simulink model "motor1"  (R2016a)
settings: Solver=ode3  StartTime=0.0  StopTime=1  MaxStep=1e-4  RelTol=1e-3
values from neighbouring files (symbols this model uses):
  D = chromosome(chromosomeProperties.populationNumber+1).gene(3).value    [HW1.m]    (also in motorModel01.m = 0.03; motorModel03.m = 8.42)
  I = chromosome(chromosomeProperties.populationNumber+1).gene(2).value    [HW1.m]    (also in motorModel01.m = 14.2; motorModel03.m = 18638)
  P = chromosome(chromosomeProperties.populationNumber+1).gene(1).value    [HW1.m]    (also in motorModel01.m = 1.35; motorModel03.m = 792.12)
libraries: simulink x1
settings Model: Creator=Minh  LastModifiedBy=Minh
settings DataIOCC: LimitDataPoints=on  SaveFormat=Array
settings DebuggingCC: UnderspecifiedInitializationDetection=Classic  MergeDetectMultiDrivingBlocksExec=none  SolverPrmCheckMsg=warning  StateNameClashWarn=warning
settings HardwareCC: ProdBitPerPointer=32  ProdLargestAtomicFloat=None  ProdIntDivRoundTo=Undefined  ProdEndianess=Unspecified  ProdWordSize=32  ProdHWDeviceType=32-bit Generic
settings ModelReferenceCC: PropagateSignalLabelsOutOfModel=off
settings ConfigComp: CovModelRefEnable=Off
settings ConfigurationSet: Description=SimMechanics 2G

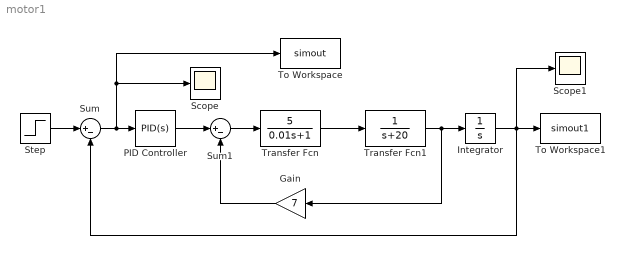
== system motor1 ==
  Gain : Gain  Gain=7
  Integrator : Integrator
  PID Controller : simulink/Continuous/PID Controller  Controller=PID  TimeDomain=Continuous-time  SampleTime=-1  IntegratorMethod=Forward Euler  FilterMethod=Forward Euler  Form=Parallel  UseFilter=on  ControllerParametersSource=internal  P=P  I=I  D=D  N=1000  InitialConditionSource=internal  InitialConditionForIntegrator=0  InitialConditionForFilter=0  ExternalReset=none  LimitOutput=off  UpperSaturationLimit=inf  LowerSaturationLimit=-inf  LinearizeAsGain=on  AntiWindupMode=none  Kb=1  TrackingMode=off  Kt=1  PParamMin=[]  PParamMax=[]  IParamMin=[]  IParamMax=[]  DParamMin=[]  DParamMax=[]  NParamMin=[]  NParamMax=[]  KbParamMin=[]  KbParamMax=[]  KtParamMin=[]  KtParamMax=[]  POutMin=[]  POutMax=[]  IOutMin=[]  IOutMax=[]  DOutMin=[]  DOutMax=[]  NOutMin=[]  NOutMax=[]  KbOutMin=[]  KbOutMax=[]  KtOutMin=[]  KtOutMax=[]  IntegratorOutMin=[]  IntegratorOutMax=[]  FilterOutMin=[]  FilterOutMax=[]  SumOutMin=[]  SumOutMax=[]  SumI1OutMin=[]  SumI1OutMax=[]  SumI2OutMin=[]  SumI2OutMax=[]  SumI3OutMin=[]  SumI3OutMax=[]  SumDOutMin=[]  SumDOutMax=[]  SaturationOutMin=[]  SaturationOutMax=[]  IntegratorContinuousStateAttributes=''  IntegratorStateMustResolveToSignalObject=off  IntegratorRTWStateStorageClass=Auto  FilterContinuousStateAttributes=''  FilterStateMustResolveToSignalObject=off  FilterRTWStateStorageClass=Auto  DifferentiatorICPrevScaledInput=0  DifferentiatorOutMin=[]  DifferentiatorOutMax=[]
  Scope : Scope
  Scope1 : Scope
  Step : Step  Time=0  SampleTime=0.001
  Sum : Sum  Inputs=|+-
  Sum1 : Sum  Inputs=|+-
  To Workspace : ToWorkspace  VariableName=simout  SampleTime=0.001
  To Workspace1 : ToWorkspace  VariableName=simout1  SampleTime=0.001
  Transfer Fcn : TransferFcn  Numerator=[5]  Denominator=[0.01 1]
  Transfer Fcn1 : TransferFcn  Denominator=[1 20]
  wires:
  Step/1 -> Sum/1
  Sum/1 -> Scope/1, To Workspace/1, PID Controller/1
  PID Controller/1 -> Sum1/1
  Sum1/1 -> Transfer Fcn/1
  Transfer Fcn/1 -> Transfer Fcn1/1
  Transfer Fcn1/1 -> Gain/1, Integrator/1
  Gain/1 -> Sum1/2
  Integrator/1 -> Scope1/1, Sum/2, To Workspace1/1
